simulink model "harness"  (R2020b)
settings: Solver=FixedStepAuto  StartTime=0.0  StopTime=2  FixedStep=0.000001  RelTol=1e-3
settings Model: Creator=GUO HUI  LastModifiedBy=GUO HUI

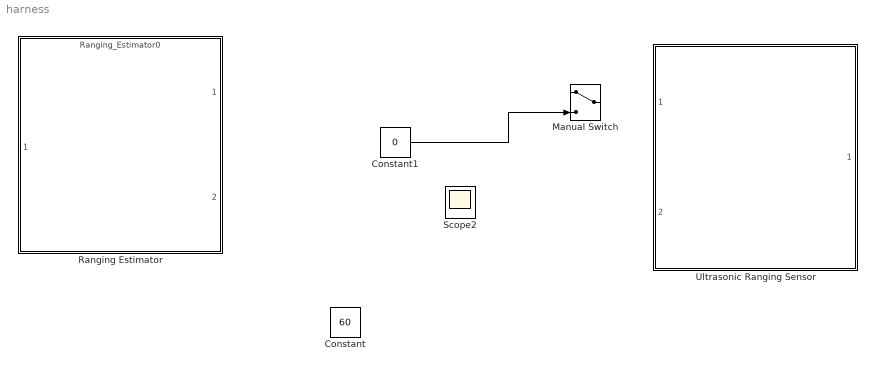
== system harness ==
  Constant : Constant  Value=60
  Constant1 : Constant  Value=0
  Manual Switch : ManualSwitch
  Ranging Estimator : ModelReference  ModelNameDialog=Ranging_Estimator0  SimulationMode=Normal  ModelReferenceVersion=1.1
  Scope2 : Scope
  Ultrasonic Ranging Sensor : Subsystem  TreatAsAtomicUnit=on  ReferencedSubsystem=Ultrasonic_Ranging_Sensor
  wires:
  Constant1/1 -> Manual Switch/2
